simulink model "lab06par01"  (R2015a)
settings: Solver=ode45  StartTime=0.0  StopTime=10.0  RelTol=1e-3
settings Model: Creator=dg  LastModifiedBy=dg

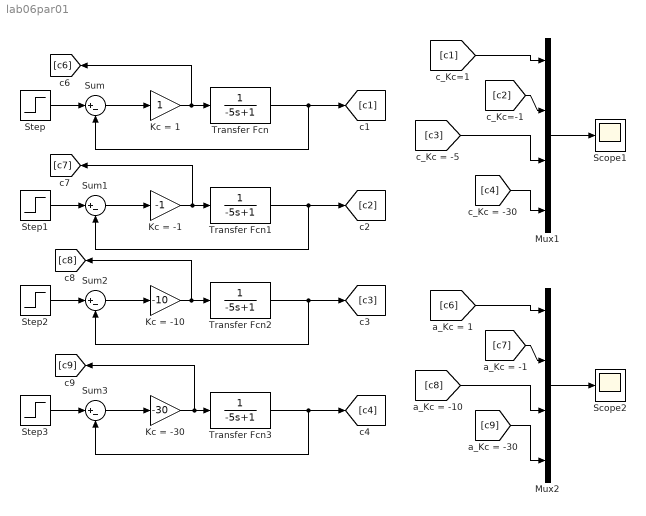
== system lab06par01 ==
  Kc = -1 : Gain  Gain=-1
  Kc = -10 : Gain  Gain=-10
  Kc = -30 : Gain  Gain=-30
  "Kc = 1 " : Gain
  Mux1 : Mux
  Mux2 : Mux
  Scope1 : Scope
      settings: ShowLegends=on  YMin=-1  YMax=1.5
  Scope2 : Scope
      settings: ShowLegends=on  YMax=10
  Step{,1..3} (4 alike) : Step  Time=0  SampleTime=0
  Sum{,1..3} (4 alike) : Sum  Inputs=|+-
  Transfer Fcn{,1..3} (4 alike) : TransferFcn  Denominator=[-5 1]
  wires:
  Step/1 -> Sum/1
  Sum/1 -> "Kc = 1 "/1
  "Kc = 1 "/1 -> [c6], Transfer Fcn/1
  Transfer Fcn/1 -> Sum/2, [c1]
  Step1/1 -> Sum1/1
  Sum1/1 -> Kc = -1/1
  Kc = -1/1 -> [c7], Transfer Fcn1/1
  Transfer Fcn1/1 -> Sum1/2, [c2]
  Step2/1 -> Sum2/1
  Sum2/1 -> Kc = -10/1
  Kc = -10/1 -> [c8], Transfer Fcn2/1
  Transfer Fcn2/1 -> Sum2/2, [c3]
  Step3/1 -> Sum3/1
  Sum3/1 -> Kc = -30/1
  Kc = -30/1 -> [c9], Transfer Fcn3/1
  Transfer Fcn3/1 -> Sum3/2, [c4]
  Mux1/1 -> Scope1/1
  [c1] -> Mux1/1
  [c2] -> Mux1/2
  [c3] -> Mux1/3
  [c4] -> Mux1/4
  Mux2/1 -> Scope2/1
  [c6] -> Mux2/1
  [c7] -> Mux2/2
  [c8] -> Mux2/3
  [c9] -> Mux2/4
